simulink model "QRD_Householder_Ex1"  (R2025a)
settings: Solver=VariableStepAuto  StartTime=0.0  StopTime=10  RelTol=1e-3
InitFcn:
  | A = single(rand(8,8));
undefined symbols (not defined in the file): major, Row, S, static_input_Convolution_Stream_Ex1, Subsystem, vsva2197, xcvc1902
libraries: aieUtilities x2, aieSolver x1, vmcUtilities x1
settings Model: Creator=sdegala  LastModifiedBy=sdegala
settings ModelReferenceCC: EnableRefExpFcnMdlSchedulingChecks=on
settings RTWCC: GPUComputeCapability=3.5

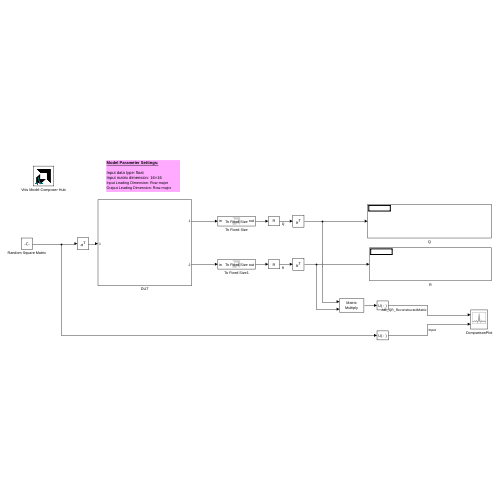
[thumbnail: Simulink's stored preview of the top-level diagram]
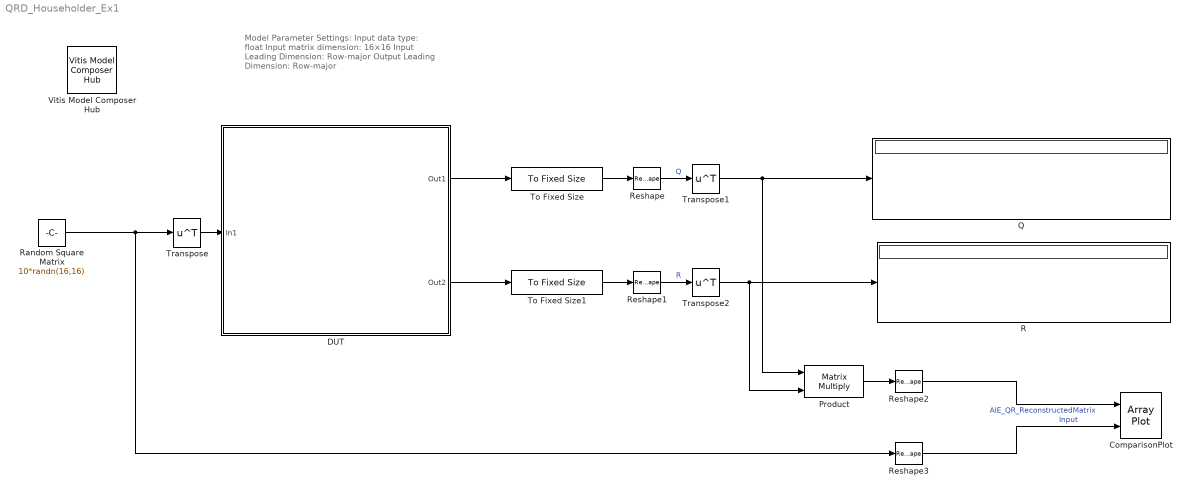
== system QRD_Householder_Ex1 ==
  note: Model Parameter Settings:
      |
      | Input data type: float
      | Input matrix dimension: 16×16
      | Input Leading Dimension: Row-major
      | Output Leading Dimension: Row-major
  ComparisonPlot : ArrayPlot  NumInputPorts=2  WindowPosition=[6.000000,6.000000,1904.000000,1097.000000,]  Visible=on  ScopeFrameLocation=window  YLimits=[-39.8468 35.4172]  ShowLegend=on
  DUT : Subsystem
  Product : Product  Multiplication=Matrix(*)
  Q : Display
  R : Display
  Random Square Matrix : Constant  Value=10*randn(16,16)  OutDataTypeStr=single  SampleTime=1
  Reshape : Reshape  OutputDimensionality=Customize  OutputDimensions=[16,16]
  Reshape1 : Reshape  OutputDimensionality=Customize  OutputDimensions=[16,16]
  Reshape2 : Reshape
  Reshape3 : Reshape
  To Fixed Size : aieUtilities/To Fixed Size  Mode=Stop simulation when input variable-size signal is not full  OutputSize=Inherit: Same as input  CopyMethod=Buffer samples to form output  HasStatusOutput=on
  To Fixed Size1 : aieUtilities/To Fixed Size  Mode=Stop simulation when input variable-size signal is not full  OutputSize=Inherit: Same as input  CopyMethod=Buffer samples to form output  HasStatusOutput=on
  Transpose : Math  Operator=transpose
  Transpose1 : Math  Operator=transpose
  Transpose2 : Math  Operator=transpose
  Vitis Model Composer Hub : vmcUtilities/Vitis Model Composer Hub  Tag=genX  CodeGeneration=off  SubsystemName=Subsystem  BlockHierPath=static_input_Convolution_Stream_Ex1/Subsystem  SubsystemType=AIENode  AIEArrayConfig=Use entire AIE array  StartColumn=1  NumberOfColumns=1  TargetDirectory=./code  exportDesign=on  analyzeDesign=off  validateDesignOnHw=off  ExportType=AI Engines  IpVendor=xilinx.com  IpLibrary=hls  IpVersion=1.0  IpHWLanguage=Verilog  AieCompilerOptions={}  AieSimulatorOptions={}  CreateTestbench=on  TestbenchStackSize=10  RunRtlSim=off  RunCSim=off  RunAieSim=off  enableSimulationTimeout=on  enableGraphIterations=on  AieSimTimeout=50000  AieGraphIterations=-1  RunAieSimProfiling=off  LaunchVitisAnalyzer=off  PlotOutput=off  RunX86Sim=off  X86SimTimeout=10  GenHwImage=off  GenLibadfXo=off  GenHwValidationCode=off  PlatformType=Not Specified  HwSystemType=Baremetal  HwValidationTarget=hw  ProjDevice=xcvc1902-vsva2197-1LP-e-S  ProjDevicePart=xcvc1902-vsva2197-1LP-e-S  AIEType=AIE  SamplePeriod=-1  ClockFrequency=200  DataPathParallelism=1  xilinxfamily=versalaicore  part=xcvc1902  speed=-1LP-e-S  package=vsva2197  directory=./netlist  testbench=off  incr_netlist=off  synthesis_tool=Vivado  clock_wrapper=Clock Enables  dbl_ovrd=According to Block Masks  dcm_input_clock_period=10  sysclk_period=10  simulink_period=1  eval_field=0  IPInfoJsonString="{\"DUTSubsystemName\":\"Subsystem\",\"AIESubsystem\":{\"SubsystemName\":\"Subsystem\",\"TargetDirectory\":\"./code\",\"AIEArrayConfig\":\"Use entire AIE array\",\"StartColumn\":\"0\",\"NumberOfColumns\":\"1\"},\"SubsystemTag\":\"AIENode\"}"  LogFileName=/tmp/CR-1250814/code/model_composer.log  NThreads=4  IPConfigFile=/tmp/vmctmp-13380004059271250980/static_input_Convolution_Stream_Ex1_ipconfig.json
  wires:
  Random Square Matrix/1 -> Transpose/1, Reshape3/1
  To Fixed Size/1 -> Reshape/1
  Reshape/1 -> Transpose1/1  "Q"
  To Fixed Size1/1 -> Reshape1/1
  Reshape1/1 -> Transpose2/1  "R"
  Product/1 -> Reshape2/1
  Reshape2/1 -> ComparisonPlot/1  "AIE_QR_ReconstructedMatrix"
  Reshape3/1 -> ComparisonPlot/2  "Input"
  DUT/1(Out1) -> To Fixed Size/1
  DUT/2(Out2) -> To Fixed Size1/1
  Transpose/1 -> DUT/1(In1)
  Transpose1/1 -> Q/1, Product/1
  Transpose2/1 -> R/1, Product/2

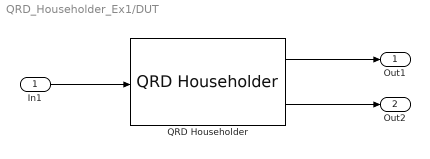
== system QRD_Householder_Ex1/DUT ==
  In1 : Inport
  QRD Householder : aieSolver/QRD Householder  AIE_VARIANT=1  data_type=float  row_dimension=16  cols_dimension=16  num_frames=1  casc_length=1  dim_a_leading=Row-major(1)  dim_q_leading=Row-major(1)  dim_r_leading=Row-major(1)  blockJsonConstraints=[]  blockJsonConstraintsInternal=[]  spec=vmc_qrd_hh.json  SerializedMaskParamNames=[]  SerializedMaskParamValues=[]  SerializedMaskParamVisibilities=[]  block_type=QRD Householder  SerializedMaskParamDataypes=uint|typename|uint|uint|uint|uint|uint|uint|uint  SerializedMaskParamEnumStrArr=0|0|0|0|0|0|Column-major(0),Row-major(1)|Column-major(0),Row-major(1)|Column-major(0),Row-major(1)  SerializedMaskParamEnumValArr=0|0|0|0|0|0|0,1|0,1|0,1  SerializedMaskParamVectorArr=0|0|0|0|0|0|0|0|0  SerializedMaskParamKeys=AIE_VARIANT|TT_DATA|TP_DIM_ROWS|TP_DIM_COLS|TP_NUM_FRAMES|TP_CASC_LEN|TP_DIM_A_LEADING|TP_DIM_Q_LEADING|TP_DIM_R_LEADING
  Out1 : Outport
  Out2 : Outport  Port=2
  wires:
  In1/1 -> QRD Householder/1
  QRD Householder/2 -> Out2/1
  QRD Householder/1 -> Out1/1
